simulink model "NLADRC"  (R2020b)
settings: Solver=VariableStepAuto  StartTime=0.0  StopTime=10.0  RelTol=1e-3
settings Model: Creator=jswl  LastModifiedBy=jswl

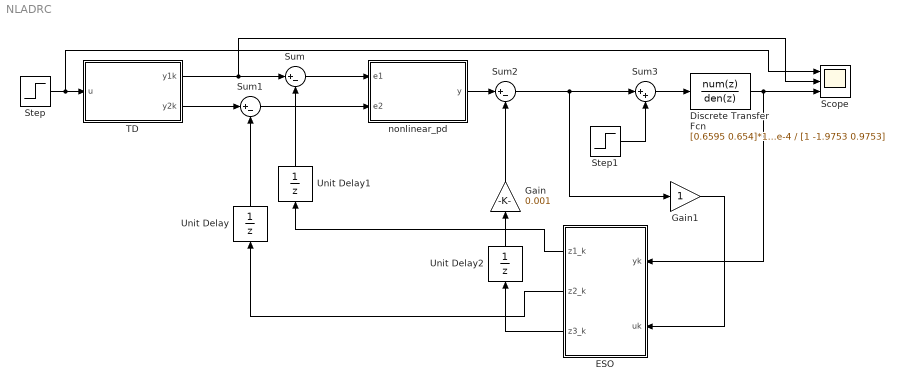
== system NLADRC ==
  Discrete Transfer Fcn : DiscreteTransferFcn  Numerator=[0.6595 0.654]*1e-4  Denominator=[1 -1.9753 0.9753]  SampleTime=0.01
  ESO : MATLAB Function  TreatAsAtomicUnit=on
  Gain : Gain  Gain=0.001
  Gain1 : Gain
  Scope : Scope  NumInputPorts=3
  Step : Step  SampleTime=0.01
  Step1 : Step  SampleTime=0.01
  Sum : Sum  Inputs=|+-
  Sum1 : Sum  Inputs=|+-
  Sum2 : Sum  Inputs=|+-
  Sum3 : Sum  Inputs=|++
  TD : MATLAB Function  TreatAsAtomicUnit=on
  Unit Delay : UnitDelay  SampleTime=0.01  HasFrameUpgradeWarning=on
  Unit Delay1 : UnitDelay  SampleTime=0.01  HasFrameUpgradeWarning=on
  Unit Delay2 : UnitDelay  SampleTime=0.01  HasFrameUpgradeWarning=on
  nonlinear_pd : MATLAB Function  TreatAsAtomicUnit=on
  wires:
  Step/1 -> TD/1(u), Scope/1
  TD/2(y2k) -> Sum1/1
  TD/1(y1k) -> Scope/2, Sum/1
  Sum/1 -> nonlinear_pd/1(e1)
  Sum1/1 -> nonlinear_pd/2(e2)
  nonlinear_pd/1(y) -> Sum2/1
  Sum2/1 -> Gain1/1, Sum3/1
  Step1/1 -> Sum3/2
  Gain1/1 -> ESO/2(uk)
  Gain/1 -> Sum2/2
  Sum3/1 -> Discrete Transfer Fcn/1
  Discrete Transfer Fcn/1 -> ESO/1(yk), Scope/3
  Unit Delay1/1 -> Sum/2
  Unit Delay/1 -> Sum1/2
  ESO/1(z1_k) -> Unit Delay1/1
  ESO/2(z2_k) -> Unit Delay/1
  ESO/3(z3_k) -> Unit Delay2/1
  Unit Delay2/1 -> Gain/1

== matlab function NLADRC/TD ==
  data: u input; y1k output; y2k output
function [y1k,y2k] = fcn(u)
persistent y1k_1 y2k_1
h=0.01;
delta=10;
if isempty(y1k_1)
    y1k_1=0;
end
 
if isempty(y2k_1)
    y2k_1=0;
end
 
y1k=y1k_1+h*y2k_1;
 
%%%%%%%%%%%%%%%%%%%%%%%%%%%%%%%%%%%%%%%%%%%%%%%hfst计算内容
d=delta*h;
d0=h*d;
y=y1k_1-u+h*y2k_1;
a0=sqrt(d*d+8*delta*abs(y));
a=0;
out1=0;
if abs(y)>d0
    a=y2k_1+(a0-d)/2*sign(y);
end
if abs(y)<=d0
    a=y2k_1+y/h;
end
if abs(a)>d
    out1=-delta*sign(a);
end
if abs(a)<=d
    out1=-delta*a/d;
end
out=out1;
%%%%%%%%%%%%%%%%%%%%%%%%%%%%%%%%%%%%%%%%%%%%
 
y2k=y2k_1+h*out;
 
y1k_1=y1k;
y2k_1=y2k;
 
y1k=y1k;
y2k=y2k;
 
end

== matlab function NLADRC/nonlinear_pd ==
  data: e1 input; y output; e2 input
function y =nonlinear_pd(e1,e2)
alfa1=0.75;
alfa2=1.5;
delta=0.02;
beta1=120;
beta2=10;
fal1=1;
fal2=1;

if abs(e1)<=delta
    fal1=e1/(delta^(1-alfa1));
end

if abs(e1)>delta
    fal1=(abs(e1))^(alfa1)*sign(e1);
end

if abs(e2)<=delta
    fal2=e2/(delta^(1-alfa2));
end

if abs(e2)>delta
    fal2=(abs(e2))^(alfa2)*sign(e2);
end

y=beta1*fal1+beta2*fal2;
end

== matlab function NLADRC/ESO ==
  settings: updateMethod=DISCRETE
  data: yk input; z1_k output; z2_k output; uk input; z3_k output
function [z1_k,z2_k,z3_k] = ESO(yk,uk)
%%参数初始化
persistent  z1_k_1 z2_k_1 z3_k_1
bata01=20;
beta02=200;
beta03=800;
b=1.4;
h=0.01;
alfa1=0.75;
alfa2=1.5;
delta=0.02;
fal1=1;
fal2=1;
if isempty(z1_k_1)
    z1_k_1=0;
end
if isempty(z2_k_1)
    z2_k_1=0;
end
if isempty(z3_k_1)
    z3_k_1=0;
end

e1=z1_k_1-yk;
z1_k=z1_k_1+h*(z2_k_1-bata01*e1);
z1_k_1=z1_k; %%迭代更新z1_k_1

%%计算fal函数
if abs(e1)<=delta
    fal1=e1/(delta^(1-alfa1));
end
if abs(e1)>delta
    fal1=(abs(e1))^(alfa1)*sign(e1);
end
if abs(e1)<=delta
    fal2=e1/(delta^(1-alfa2));
end
if abs(e1)>delta
    fal2=(abs(e1))^(alfa2)*sign(e1);
end

z2_k=z2_k_1+h*(z3_k_1-beta02*fal1+b*uk);
z2_k_1=z2_k;%%迭代更新z2_k_1

z3_k=z3_k_1-h*beta03*fal2;
z3_k_1=z3_k;%%迭代更新z3_k_1

end
